simulink model "untitled"  (R2015a)
settings: Solver=ode3  StartTime=0.0  StopTime=10.0  RelTol=1e-3
settings Model: Creator=Panoply  LastModifiedBy=Panoply
settings OptimizationCC: OptimizeModelRefInitCode=on  LifeSpan=1  MaxStackSize=64
settings HardwareCC: ProdLargestAtomicInteger=Long  ProdLargestAtomicFloat=Double  ProdEndianess=LittleEndian  ProdHWDeviceType=ARM Compatible->ARM Cortex
settings RTWCC: SystemTargetFile=ert.tlc  GenCodeOnly=on  TemplateMakefile=ert_default_tmf  Description=Embedded Coder  Toolchain=GNU Tools for ARM Embedded Processors
settings CodeAppCC: IgnoreCustomStorageClasses=off
settings ERTTargetCC: TargetLangStandard=C99 (ISO)  ParMdlRefBuildCompliant=on  CompOptLevelCompliant=on  ConcurrentExecutionCompliant=on  ERTFirstTimeCompliant=on  IncludeFileDelimiter=UseQuote  SupportVariableSizeSignals=off  ModelStepFunctionPrototypeControlCompliant=on  CPPClassGenCompliant=on  InlinedParameterPlacement=Hierarchical  GlobalDataDefinition=InSourceFile  GlobalDataReference=InSourceFile  ERTFilePackagingFormat=Compact  SuppressUnreachableDefaultCases=on

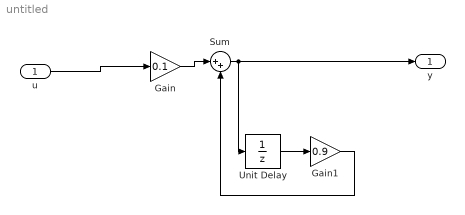
== system untitled ==
  u : Inport
  Gain : Gain  Gain=0.1
  Gain1 : Gain  Gain=0.9
  Sum : Sum  Inputs=|++
  Unit Delay : UnitDelay  SampleTime=-1
  y : Outport
  wires:
  Sum/1 -> y/1, Unit Delay/1
  Unit Delay/1 -> Gain1/1
  Gain1/1 -> Sum/2
  Gain/1 -> Sum/1
  u/1 -> Gain/1
